simulink model "pendule_inv_etu"  (R2017a)
settings: Solver=VariableStepAuto  StartTime=0.0  StopTime=10.0  RelTol=1e-3
values from neighbouring files (symbols this model uses):
  K = [30 10]    [exemple_test_pendule_inv.m]    (also in exemple_test_pendule_inv_capteur.m = [10 1]; exemple_test_pendule_inv_echant.m)
  x0 = [pi/10 0]    [exemple_test_pendule_inv.m]    (also in exemple_test_pendule_inv_capteur.m = [pi/20 0]; exemple_test_pendule_inv_echant.m = [pi/20 0])
settings Model: Creator=aandre2  LastModifiedBy=aandre2

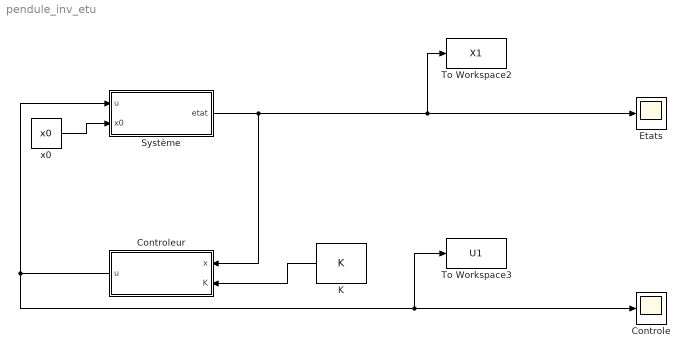
== system pendule_inv_etu ==
  Controle : Scope
  Controleur : Subsystem
  Etats : Scope
  K : Constant  Value=K
  Système : Subsystem
  To Workspace2 : ToWorkspace  VariableName=X1  SaveFormat=Timeseries  SampleTime=-1
  To Workspace3 : ToWorkspace  VariableName=U1  SaveFormat=Timeseries  SampleTime=-1
  x0 : Constant  Value=x0
  wires:
  Système/1(etat) -> Controleur/1(x), To Workspace2/1, Etats/1
  Controleur/1(u) -> To Workspace3/1, Controle/1, Système/1(u)
  K/1 -> Controleur/2(K)
  x0/1 -> Système/2(x0)

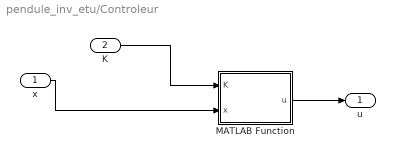
== system pendule_inv_etu/Controleur ==
  x : Inport
  K : Inport  Port=2
  MATLAB Function : MATLAB Function  TreatAsAtomicUnit=on
  u : Outport
  wires:
  x/1 -> MATLAB Function/2(x)
  MATLAB Function/1(u) -> u/1
  K/1 -> MATLAB Function/1(K)

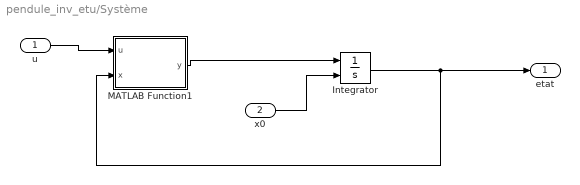
== system pendule_inv_etu/Système ==
  u : Inport
  x0 : Inport  Port=2
  Integrator : Integrator  InitialConditionSource=external
  MATLAB Function1 : MATLAB Function  TreatAsAtomicUnit=on
  etat : Outport  PortDimensions=2
  wires:
  u/1 -> MATLAB Function1/1(u)
  MATLAB Function1/1(y) -> Integrator/1
  Integrator/1 -> MATLAB Function1/2(x), etat/1
  x0/1 -> Integrator/2

== matlab function pendule_inv_etu/Controleur/MATLAB Function ==
  data: K input; x input; u output
function u = fcn(K, x)
xe = [0 0];
ue= 0;
u = ue + K(1) * (x(1) - xe(1)) + K(2)*(x(2) -xe(2)) ;

== matlab function pendule_inv_etu/Système/MATLAB Function1 ==
  data: u input; y output; x input
function y = fcn(u, x)
g = 9.81;
l = 10;
y = [0 0];
y(1) = x(2);
y(2) = g/l*sin(x(1))-cos(x(1))*u/l;
